simulink model "test2"  (Simulink 8.4)
settings: Solver=ode45  SolverMode=SingleTasking  StartTime=0.0  StopTime=10.0  RelTol=1e-3
settings Model: Creator=GM  LastModifiedBy=GM  CovMetricSettings=dwe  CovHtmlReporting=off  covSaveCumulativeToWorkspaceVar=off  CovSaveSingleToWorkspaceVar=off  CovExternalEMLEnable=on
settings DataIOCC: LimitDataPoints=off  SaveFormat=StructureWithTime  SignalLoggingSaveFormat=Dataset
settings OptimizationCC: ExpressionDepthLimit=128
settings DebuggingCC: UnderspecifiedInitializationDetection=Simplified  MergeDetectMultiDrivingBlocksExec=error  SolverPrmCheckMsg=none  FcnCallInpInsideContextMsg=EnableAllAsWarning  FrameProcessingCompatibilityMsg=error  StateNameClashWarn=none  SFUnexpectedBacktrackingDiag=error  SFNoUnconditionalDefaultTransitionDiag=error
settings HardwareCC: ProdBitPerPointer=64  ProdLargestAtomicFloat=Float  ProdIntDivRoundTo=Zero  ProdEndianess=LittleEndian  ProdHWDeviceType=Specified
settings GRTTargetCC: TargetLangStandard=C99 (ISO)  GeneratePreprocessorConditionals=Use local settings

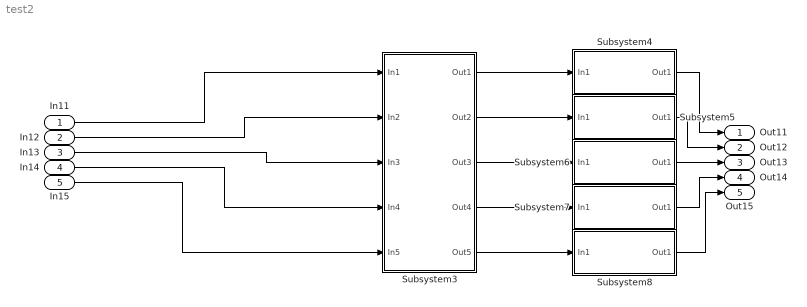
== system test2 ==
  In11 : Inport
  In12 : Inport  Port=2
  In13 : Inport  Port=3
  In14 : Inport  Port=4
  In15 : Inport  Port=5
  Subsystem3 : Subsystem
  Subsystem4 : Subsystem
      settings: AttributesFormatString=|
      | %<BlockType>
      | %<Handle>
  Subsystem5 : Subsystem
  Subsystem6 : Subsystem
  Subsystem7 : Subsystem
  Subsystem8 : Subsystem
  Out11 : Outport
  Out12 : Outport  Port=2
  Out13 : Outport  Port=3
  Out14 : Outport  Port=4
  Out15 : Outport  Port=5
  wires:
  Subsystem3/1(Out1) -> Subsystem4/1(In1)
  Subsystem3/2(Out2) -> Subsystem5/1(In1)
  Subsystem3/3(Out3) -> Subsystem6/1(In1)
  Subsystem3/4(Out4) -> Subsystem7/1(In1)
  Subsystem3/5(Out5) -> Subsystem8/1(In1)
  Subsystem4/1(Out1) -> Out11/1
  Subsystem5/1(Out1) -> Out12/1
  Subsystem6/1(Out1) -> Out13/1
  Subsystem7/1(Out1) -> Out14/1
  Subsystem8/1(Out1) -> Out15/1
  In13/1 -> Subsystem3/3(In3)
  In12/1 -> Subsystem3/2(In2)
  In14/1 -> Subsystem3/4(In4)
  In11/1 -> Subsystem3/1(In1)
  In15/1 -> Subsystem3/5(In5)

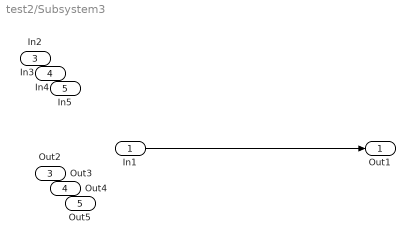
== system test2/Subsystem3 ==
  In1 : Inport
  In2 : Inport  Port=2
  In3 : Inport  Port=3
  In4 : Inport  Port=4
  In5 : Inport  Port=5
  Out1 : Outport
  Out2 : Outport  Port=2
  Out3 : Outport  Port=3
  Out4 : Outport  Port=4
  Out5 : Outport  Port=5
  wires:
  In1/1 -> Out1/1

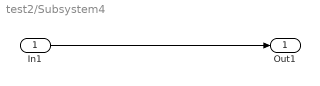
== system test2/Subsystem4 ==
  In1 : Inport
  Out1 : Outport
  wires:
  In1/1 -> Out1/1

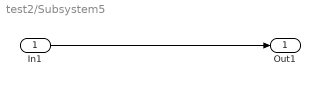
== system test2/Subsystem5 ==
  In1 : Inport
  Out1 : Outport
  wires:
  In1/1 -> Out1/1

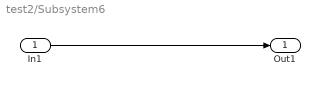
== system test2/Subsystem6 ==
  In1 : Inport
  Out1 : Outport
  wires:
  In1/1 -> Out1/1

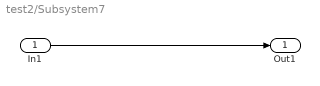
== system test2/Subsystem7 ==
  In1 : Inport
  Out1 : Outport
  wires:
  In1/1 -> Out1/1

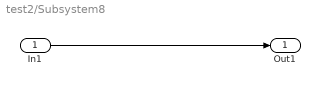
== system test2/Subsystem8 ==
  In1 : Inport
  Out1 : Outport
  wires:
  In1/1 -> Out1/1
